simulink library "powerlib_modelsV2"  (Simulink 6.0)
settings: Solver=ode45  SolverMode=SingleTasking  StartTime=0.0  StopTime=10.0  RelTol=1e-3
values from neighbouring files (symbols this model uses):
  Ts = get(handles.edit1,'string')    [powergui.m]
undefined symbols (not defined in the file or in its folder): A, Ac, B, Bc, C, Cc, Cs, Current, damp, Dc, Dd, DiscIntNeverNeededParam, dref, dwo, exc, F, fb, gate, GH, GHd, GI, GId, GL, GLd, H, HT, hyd, ib, ib2, io, isfinite, j, K, Kd, Kg, L, Lad, Laq, lim, LIM, Ll, Llfd, Llkd, Llkq1, Llkq2, Llr, Lls, LowerFlux, N, N2, Nb, Nb2, nb_arm, p, Par_HarmoA_pu, Par_HarmoB_pu, Par_Timing_Harmo, Par_Timing_Variation, Par_Vps, Pb ... (+57)
libraries: powerlib_extras x14
(part 2 of 11)

== system powerlib_modelsV2/Discrete ==
  3_Phase_Prog_Source : Subsystem  mask(Discrete 3-phase Programmable Source){Par_Vps_LLrms=[1.01 -20  60], VariationEntity=Amplitude, VariationType=Step, VariationStep=-0.5, VariationRate=10, VariationMag=0.3, VariationFreq=2, Par_Timing_Variation=[0.1 1.2], SinglePhase=off, Yampli=[1 0.8 1.2 1.0], Xtime=[0 0.1 0.15 0.2], HarmonicGeneration=off, Par_HarmoA_pu=[3 0.2 -25 0], Par_HarmoB_pu=[2 0.15 35 2], Par_Timing_Harmo=[0.05  3], Ts=50e-6}
      mask prompts: Par_Vps_LLrms "Positive-sequence: [ Amplitude  Phase(degrees)   Freq. (Hz) ]"; VariationEntity "Time variation of:"; VariationType "Type of variation:"; VariationStep "Step magnitude:"; VariationRate "Rate of change (value/s):"; VariationMag "Amplitude of the modulation:"; VariationFreq "Frequency of the modulation(Hz):"; Par_Timing_Variation "Variation timing (s) : [ Start   End ]"; SinglePhase "1-phase only"; Yampli "Amplitude values:"; Xtime "Time values:"; HarmonicGeneration "Harmonic generation:"; Par_HarmoA_pu "A:  [ Order(n)   Amplitude  Phase(degrees)  Seq(0, 1 or 2) ]"; Par_HarmoB_pu "B:  [ Order(n)   Amplitude  Phase(degrees)  Seq(0, 1 or 2) ]"; Par_Timing_Harmo "Harmonic timing (s) : [ Start   End ]"; Ts "Sample time:"
      mask help: Use this discrete block to generate a set of three-phase sinusoidal voltages or currents a, b and c. Time variation for the amplitude, phase and frequency of the fundamental can be pre-programmed. In addition, two harmonics can be surimposed on the fundamental.
      mask init:
      | % Conversion of pos. seq.amplitude from Ph-Ph rms voltage to Ph-G peak
      | Par_Vps=Par_Vps_LLrms;
      | Par_Vps(1)=Par_Vps(1)*sqrt(2/3);
      | Mag_Vps=Par_Vps(1);
      | Phase_Vps=Par_Vps(2);
      | Freq_Vps=Par_Vps(3);
      | % Conversion of harmonic amplitudes from pu to Ph-G peak volt
      | Par_HarmoA=Par_HarmoA_pu;
      | Par_HarmoB=Par_HarmoB_pu;
      | Par_HarmoA(2)=Par_HarmoA(2)*Mag_Vps;
      | Par_HarmoB(2)=Par_HarmoB(2)*Mag_Vps;
      | % Conversion of amplitude variation from pu to Ph-G peak volt
      | if VariationEntity==2
      | 	VariationStep=VariationStep*Mag_Vps;
      | 	VariationRate=VariationRate*Mag_Vps;
      | 	VariationMag=VariationMag*Mag_Vps;
      | 	Yampli=Yampli*Mag_Vps;
      | end
      | 
      | Ton_Variation=Par_Timing_Variation(1);
      | Toff_Variation=Par_Timing_Variation(2);
      | n_HarmoA=Par_HarmoA(1);
      | Mag_HarmoA=Par_HarmoA(2);
      | Phase_HarmoA=Par_HarmoA(3);
      | Seq_HarmoA=Par_HarmoA(4);
      | if n_HarmoA==0
      |     Phase_HarmoA=90;
      |     Seq_HarmoA=0;
      | end
      | n_HarmoB=Par_HarmoB(1);
      | Mag_HarmoB=Par_HarmoB(2);
      | Phase_HarmoB=Par_HarmoB(3);
      | Seq_HarmoB=Par_HarmoB(4);
      | if n_HarmoB==0
      |     Phase_HarmoB=90;
      |     Seq_HarmoB=0;
      | end
      | Ton_Harmo=Par_Timing_Harmo(1);
      | Toff_Harmo=Par_Timing_Harmo(2);
      | if Xtime(1)~=0,
      | Xtime=[0 Xtime];
      | Yampli=[0 Yampli];
      | end
      | n=length(Xtime); vec_dt= [Xtime,0] - [0,Xtime] ; vec_dt=vec_dt(2:n);
      mask StyleString: edit,popup(None|Amplitude|Phase|Frequency),popup(Step|Ramp|Modulation|Table of time-amplitude pairs),edit,edit,edit,edit,edit,checkbox,edit,edit,checkbox,edit,edit,edit,edit
      mask CallbackString: |parametres=get_param(gcb,'MaskValues');p2=parametres{2};p3=parametres{3};p12=parametres{12};if strcmp(p3,'Step');param4='on';param5='off';param6='off';param7='off';param8='on';param9='off';param10='off';param11='off';elseif strcmp(p3,'Ramp');param4='off';param5='on';param6='off';param7='off';param8='on';param9='off';param10='off';param11='off';elseif strcmp(p3,'Modulation');param4='off';param5='off';param6='on';param7='on';param8='on';param9='off';param10='off';param11='off';else;param4='off';param5='off';param6='off';param7='off';param8='off';param9='on';param10='on';param11='on';end;if strcmp(p2,'None');param3='off';param4='off';param5='off';param6='off';param7='off';param8='off';param9='off';param10='off';param11='off';else;param3='on';end;if strcmp(p12,'on');param13='on';param14='on';param15='on';else;param13='off';param14='off';param15='off';end;visible={'on','on',param3,param4,param5,param6,param7,param8,param9,param10,param11,'on',param13,param14,param15,'on'};set_param(gcb,'MaskVisibilities',visible)|parametres=get_param(gcb,'MaskValues');p2=parametres{2};p3=parametres{3};p12=parametres{12};if strcmp(p3,'Step');param4='on';param5='off';param6='off';param7='off';param8='on';param9='off';param10='off';param11='off';elseif strcmp(p3,'Ramp');param4='off';param5='on';param6='off';param7='off';param8='on';param9='off';param10='off';param11='off';elseif strcmp(p3,'Modulation');param4='off';param5='off';param6='on';param7='on';param8='on';param9='off';param10='off';param11='off';else;param4='off';param5='off';param6='off';param7='off';param8='off';param9='on';param10='on';param11='on';end;if strcmp(p2,'None');param3='off';param4='off';param5='off';param6='off';param7='off';param8='off';param9='off';param10='off';param11='off';else;param3='on';end;if strcmp(p12,'on');param13='on';param14='on';param15='on';else;param13='off';param14='off';param15='off';end;visible={'on','on',param3,param4,param5,param6,param7,param8,param9,param10,param11,'on',param13,param14,param15,'on'};set_param(gcb,'MaskVisibilities',visible)|||||||||parametres=get_param(gcb,'MaskValues');p2=parametres{2};p3=parametres{3};p12=parametres{12};if strcmp(p3,'Step');param4='on';param5='off';param6='off';param7='off';param8='on';param9='off';param10='off';param11='off';elseif strcmp(p3,'Ramp');param4='off';param5='on';param6='off';param7='off';param8='on';param9='off';param10='off';param11='off';elseif strcmp(p3,'Modulation');param4='off';param5='off';param6='on';param7='on';param8='on';param9='off';param10='off';param11='off';else;param4='off';param5='off';param6='off';param7='off';param8='off';param9='on';param10='on';param11='on';end;if strcmp(p2,'None');param3='off';param4='off';param5='off';param6='off';param7='off';param8='off';param9='off';param10='off';param11='off';else;param3='on';end;if strcmp(p12,'on');param13='on';param14='on';param15='on';else;param13='off';param14='off';param15='off';end;visible={'on','on',param3,param4,param5,param6,param7,param8,param9,param10,param11,'on',param13,param14,param15,'on'};set_param(gcb,'MaskVisibilities',visible)||||
  3_phase_source : Subsystem  mask{A=1, P=0, F=60, Ts=0}
      mask prompts: A "Amplitude"; P "Phase (of phase A)"; F "Frequency"; Ts "Sample Time"
  Dynamic_Load : Subsystem  mask(Discrete 3-Phase Dynamic Load ){Vfnom=[ 500e3 60 ], PQ_0=[ 50e6 25e6]*0.8504^2, V0=[0.8504  -41.9 ], PQext=off, n=[1 2], Tpq=[0  0  0  0], Vmin=0.7, Reserved=0, Ts=Ts}
      mask prompts: Vfnom "Nominal L-L voltage and freqency  [Vn(Vrms) fn(Hz)]:"; PQ_0 "Active & reactive power at initial voltage [Po(W) Qo(var)]:"; V0 "Initial positive-sequence voltage Vo [Mag(pu) Phase (deg.)]:"; PQext "External control of PQ"; n "Parameters [ np  nq ]:"; Tpq "Time constants [Tp1 Tp2 Tq1 Tq2]  (s):"; Vmin "Minimum voltage Vmin (pu):"; Ts "Sample time (s):"
      mask help:
      | This block implements a three-phase, three-wire dynamic load whose active  power P and reactive power Q vary as function of positive-sequence voltage. Negative- and zero-sequence currents are not simulated. The three load currents are therefore balanced, even under unbalanced load voltage conditions.
      |
      |   If V>Vmin, P and Q vary as follows:
      |        P=Po*(V/Vo)^np*(1+Tp1s)/(1+Tp2s)
      |        Q=Qo*(V/Vo)^nq*(1+Tq1s)/(1+Tq2s)
      | where:
      | Po, Qo : Active and reactive powers at specified voltage Vo
      |   V :        Positive-sequence voltage
      |   Vmin :  Minimum voltage below which load impedance
      |                is kept constant (np=nq=2)
      | np,nq :    Exponents (usually comprised between 1 and 3)
      |                controlling the nature of the load.
      | Tp1,Tp2 : Time constants controlling the dynamics of P
      | Tq1,Tq2 : Time constants controlling the dynamics of Q
      |
      | For example, specify  np=nq=1 for a constant current load; np=nq=2  for a  constant impedance load.
      |
      | Check 'External control of PQ'  to control power from a vectorized signal  [P Q] connected to input  4.
      | The m output returns a vector of 3 signals [V(pu) P(W) Q (var)].
      mask init: same as powerlib_modelsV2/Continuous/Dynamic_Load
      mask CallbackString: |||parametres=get_param(gcb,'MaskValues');p4=parametres{4};if strcmp(p4,'on');param5='off';param6='off';param7='off';else ;param5='on';param6='on';param7='on';end;visible={'on','on','on','on',param5,param6,param7,'on','on'};set_param(gcb,'MaskVisibilities',visible)|||||
  Excitation_System : Subsystem  mask(Discrete Excitation System){tr=tr, reg=reg, exc=exc, tgr=tgr, damp=damp, sat=sat, lim=lim, v0=v0, Ts=50e-6}
      mask prompts: tr "Low-pass filter time constant Tr(s):"; reg "Regulator gain and time constant [ Ka()  Ta(s) ]:"; exc "Exciter  [ Ke()  Te(s) ]:"; tgr "Transient gain reduction [ Tb(s)  Tc(s) ]:"; damp "Damping filter gain and time constant  [ Kf()  Tf(s)  ]:"; sat "Field saturation parameters [ A, B ]:"; lim "Regulator output limits and gain [ Efmin, Efmax (p.u.), Kp() ]:"; v0 "Initial values of terminal voltage  and field voltage [ Vt0 (pu) Vf0(pu) ] :"; Ts "Sample time:"
      mask help:
      | Implements an discrete IEEE type 1 synchronous machine voltage regulator combined to an exciter. This block uses the dq components of terminal voltage (Synchronous Machine block, measurement ouputs 9 and 10).
      |
      | 1st input: desired stator terminal voltage (p.u.);
      | 2nd input: vd component of the terminal voltage (p.u.);
      | 3rd input: vq component of the terminal voltage (p.u.);
      | 4th input: stabilization voltage from user-supplied
      |                  power system stabilizer (p.u.);
      |
      | output: field voltage vfd to be applied to the
      |              Synchronous Machine block's 2nd input (p.u.).
      mask init:
      | ka=reg(1);ta=reg(2);ke=exc(1);te=exc(2);tb=tgr(1);tc=tgr(2);kf=damp(1);tf=damp(2);efmin=lim(1);efmax=lim(2);a=sat(1);b=sat(2);kp=lim(3);
      | if te==0,
      | te=1e-6;
      | end
      mask Help: web(psbhelp);
  GTO-IGBT Bridge : Subsystem  mask(GTO & IGBT Bridge Logic){nb_arm=3, Tf=0, Tt=0, Cs=Inf, VFs=[0 0], Rsw=1, Ts=1}
      mask prompts: nb_arm "Number of bridge arms (1,2 or 3)"; Tf "Curent 10% fall time Tf (s) :"; Tt "Current tail time Tt (s) :"; Cs "Snubber Capacitance Cs (F):"; VFs "Forward Voltages [ Vf  Vfd ]"; Rsw "Device resistance"; Ts "Time step Ts (s) :"
      mask help:
      | Generates the switch status ( 0 or 1) and the tail currents for a forced-commutated two- level bridge using GTO/Diode or IGBT/Diode pairs.
      | Specify  3 arms (6 switches) for 3 phase bridge, 2 arms for 4 switches, or 1 arm.
      | To turn-off the tail current, specify Tf=0 and Tt=0.
      mask init:
      | Vf=VFs(1);
      | Vfd=VFs(2);
      | nb_switch=nb_arm*2;
      | if nb_arm==1,
      |    Selec_Diode=[2 1];
      | elseif nb_arm==2,
      |    Selec_Diode=[2 1 4 3];
      | elseif nb_arm==3,
      |    Selec_Diode=[2 1 4 3 6 5];
      | end
  HTG : Subsystem  mask(Discrete Hydraulic Turbine and Governor){sm=sm, gate=gate, reg=reg, hyd=hyd, dref=dref, po=po, Ts=50e-6}
      mask prompts: sm "Servo-motor [ Ka()  Ta(sec) ]:"; gate "Gate opening limits [ gmin,gmax(pu)    vgmin,vgmax(pu/s) ]:"; reg "Permanent droop and regulator  [ Rp() Kp() Ki() Kd() Td(s) ]:"; hyd "Hydraulic turbine [ beta()  Tw(sec) ]:"; dref "Droop reference (0=power error, 1=gate opening):"; po "Initial mechanical power (pu):"; Ts "Sample time:"
      mask help:
      | Implements a discrete hydraulic turbine combined to a discrete PID governor system.
      |
      | 1st input: desired speed (p.u.);
      | 2nd input: desired electrical power (p.u.);
      | 3rd input: synchronous machine's actual speed (p.u., measurement output 13 of SM block);
      | 4th input: synchronous machine's actual electrical power (p.u., measurement output 14 of SM block);
      | 5th input: synchronous machine's actual speed deviation with respect to nominal (%, measurement output 15 of SM block);
      |
      | 1st output: mechanical power to be applied to the Synchronous Machine block's 1st input (p.u.);
      | 2nd output: gate opening (p.u.).
      mask init:
      | ka=sm(1);ta=sm(2);gmin=gate(1);gmax=gate(2);vgmin=gate(3);vgmax=gate(4);Rp=reg(1);kp=reg(2);ki=reg(3);kd=reg(4);td=reg(5);beta=hyd(1);tw=hyd(2);go=po*(gmax-gmin);
      mask Help: web(psbhelp);
  Impedance Measurement : Subsystem
      mask Type: Impedance Measurement model
      mask Description: The impedance Measurement block injects a null current in the circuit.
  MBPSS : Subsystem  mask(MB-PSS ){OperationMode=Detailed settings, Kg=Kg, GL=GL, GI=GI, GH=GH, GLd=GLd, TcLF=TcLF, GId=GId, TcIF=TcIF, GHd=GHd, TcHF=TcHF, LIM=LIM, Plot_On=off, MagdB_On=off, FreqRange=logspace(-2,2,500), Ts=50e-6}
      mask prompts: OperationMode "Mode of operation:"; Kg "Global gain:"; GL "Low frequency band: [ FL(Hz), KL ]"; GI "Intermediate frequency band: [ FI(Hz), KI ]"; GH "High frequency band: [ FH(Hz), KH ]"; GLd "Low frequency gains: [ KL1, KL2, KL ]"; TcLF "Low frequency  time constants (s):"; GId "Intermediate frequency gains: [ KI1, KI2, KI ]"; TcIF "Intermediate frequency time constants (s):"; GHd "High frequency gains: [ KH1, KH2, KH ]"; TcHF "High frequency time constants (s):"; LIM "Signals Limits(VLmax,VImax,VHmax,VSmax)"; Plot_On "Plot frequency response"; MagdB_On "Magnitude in dB"; FreqRange "Frequency range (Hz):"
      mask help:
      | This block implements a Multi-band Power System Stabilizer (MB-PSS). Two operation modes are available: Detailed setting and simplified setting (IEEE Std 421.5).
      |
      | Input (dw): Synchronous machine speed deviation with respect to nominal (pu).
      | Output: stabilization voltage (pu).
      |
      | Note:
      | When "Detailed settings" is used, the low(L)-, intermediate(I)- and high(H)-frequency time constants must be given in the following order:
      | Tx1 to Tx12 followed by Kx11 and Kx17 (where x=L, I or H). Look under mask to see in which transfer functions these time constants are used.
      mask init:
      | Detailed=0;
      | if OperationMode==2,
      | Detailed=1;
      | Kg=1;
      | KL1=GLd(1);KL2=GLd(:,2);KL=GLd(3);
      | TL1=TcLF(1);TL2=TcLF(2);TL3=TcLF(3);TL4=TcLF(4);
      | TL5=TcLF(5);TL6=TcLF(6);TL7=TcLF(7);TL8=TcLF(8);
      | TL9=TcLF(9);TL10=TcLF(10);TL11=TcLF(11);TL12=TcLF(12);
      | KL11=TcLF(13);KL17=TcLF(14);
      | KI1=GId(1);KI2=GId(:,2);KI=GId(3);
      | TI1=TcIF(1);TI2=TcIF(2);TI3=TcIF(3);TI4=TcIF(4);
      | TI5=TcIF(5);TI6=TcIF(6);TI7=TcIF(7);TI8=TcIF(8);
      | TI9=TcIF(9);TI10=TcIF(10);TI11=TcIF(11);TI12=TcIF(12);
      | KI11=TcIF(13);KI17=TcIF(14);
      | KH1=GHd(1);KH2=GHd(:,2);KH=GHd(3);
      | TH1=TcHF(1);TH2=TcHF(2);TH3=TcHF(3);TH4=TcHF(4);
      | TH5=TcHF(5);TH6=TcHF(6);TH7=TcHF(7);TH8=TcHF(8);
      | TH9=TcHF(9);TH10=TcHF(10);TH11=TcHF(11);TH12=TcHF(12);
      | KH11=TcHF(13);KH17=TcHF(14);
      | else
      | %
      | R=1.2;K=(R*R+R)/(R*R-2*R+1);KL1=K;KL2=K;KI1=K;KI2=K;KH1=K;KH2=K;
      | TL2=1/(2*pi*GL(1)*sqrt(R));KL=GL(2);TL1=TL2/R;TL7=TL2;TL8=TL7*R;
      | %
      | TI2=1/(2*pi*GI(1)*sqrt(R));KI=GI(2);TI1=TI2/R;TI7=TI2;TI8=TI7*R;
      | TH2=1/(2*pi*GH(1)*sqrt(R));KH=GH(2);TH1=TH2/R;TH7=TH2;TH8=TH7*R;
      | %
      | TL3=0;TL4=0;TL5=0;TL6=0;TL9=0;TL10=0;TL11=0;TL12=0;
      | TI3=0;TI4=0;TI5=0;TI6=0;TI9=0;TI10=0;TI11=0;TI12=0;
      | TH3=0;TH4=0;TH5=0;TH6=0;TH9=0;TH10=0;TH11=0;TH12=0;
      | KL11=1;KL17=1;KI11=1;KI17=1;KH11=1;KH17=1;
      | end
      | LIM_VL=LIM(1);LIM_VI=LIM(2);LIM_VH=LIM(3);LIM_VS=LIM(4);
      | %
      | % LF Transfer function
      | numLF1=[TL1 KL11];
      | denLF1=[TL2 1];
      | sysLF1=tf(numLF1,denLF1);
      | numLF2=[TL3 1];
      | denLF2=[TL4 1];
      | sysLF2=tf(numLF2,denLF2);
      | numLF3=[TL5 1];
      | denLF3=[TL6 1];
      | sysLF3=tf(numLF3,denLF3);
      | numLF4=[TL7 KL17];
      | denLF4=[TL8 1];
      | sysLF4=tf(numLF4,denLF4);
      | numLF5=[TL9 1];
      | denLF5=[TL10 1];
      | sysLF5=tf(numLF5,denLF5);
      | numLF6=[TL11 1];
      | denLF6=[TL12 1];
      | sysLF6=tf(numLF6,denLF6);
      | %
      | sysLF=Kg*KL*((KL1*sysLF1*sysLF2*sysLF3) - (KL2*sysLF4*sysLF5*sysLF6));
      | %
      | %
      | % IF transfer function
      | numIF1=[TI1 KI11];
      | denIF1=[TI2 1];
      | sysIF1=tf(numIF1,denIF1);
      | numIF2=[TI3 1];
      | denIF2=[TI4 1];
      | sysIF2=tf(numIF2,denIF2);
      | numIF3=[TI5 1];
      | denIF3=[TI6 1];
      | sysIF3=tf(numIF3,denIF3);
      | numIF4=[TI7 KI17];
      | denIF4=[TI8 1];
      | sysIF4=tf(numIF4,denIF4);
      | numIF5=[TI9 1];
      | denIF5=[TI10 1];
      | sysIF5=tf(numIF5,denIF5);
      | numIF6=[TI11 1];
      | denIF6=[TI12 1];
      | sysIF6=tf(numIF6,denIF6);
      | %
      | sysIF=Kg*KI*((KI1*sysIF1*sysIF2*sysIF3) - (KI2*sysIF4*sysIF5*sysIF6));
      | %
      | %
      | % HF transfer function
      | numHF1=[TH1 KH11];
      | denHF1=[TH2 1];
      | sysHF1=tf(numHF1,denHF1);
      | numHF2=[TH3 1];
      | denHF2=[TH4 1];
      | sysHF2=tf(numHF2,denHF2);
      | numHF3=[TH5 1];
      | denHF3=[TH6 1];
      | sysHF3=tf(numHF3,denHF3);
      | numHF4=[TH7 KH17];
      | denHF4=[TH8 1];
      | sysHF4=tf(numHF4,denHF4);
      | numHF5=[TH9 1];
      | denHF5=[TH10 1];
      | sysHF5=tf(numHF5,denHF5);
      | numHF6=[TH11 1];
      | denHF6=[TH12 1];
      | sysHF6=tf(numHF6,denHF6);
      | %
      | sysHF=Kg*KH*((KH1*sysHF1*sysHF2*sysHF3) - (KH2*sysHF4*sysHF5*sysHF6));
      | %
      | %
      | % Input filter LIF
      | numLIFin=[1.759e-3 1];
      | denLIFin=[1.2739e-4 1.7823e-2 1];
      | sysLIFin=tf(numLIFin,denLIFin);
      | % Input filter HF
      | numHFin=[80 0 0];
      | denHFin=[1 82 161 80];
      | sysHFin=tf(numHFin,denHFin);
      | %
      | % Global transfer function:
      | sysL=sysLIFin*sysLF;
      | sysI=sysLIFin*sysIF;
      | sysH=sysHFin*sysHF;
      | sysG=sysL+sysI + sysH;
      | %
      | % Plot frequency response:
      | if Plot_On==1,
      |     w=2*pi*FreqRange;
      |     [MagL,PhaseL]=bode(sysL,w);
      |     [MagI,PhaseI]=bode(sysI,w);
      |     [MagH,PhaseH]=bode(sysH,w);
      |     [MagG,PhaseG]=bode(sysG,w);
      |     subplot(2,1,1)
      |      if  MagdB_On==1,
      |         YL= 20*log10(squeeze(MagL)) ;
      |         YI= 20*log10(squeeze(MagI)) ;
      |         YH= 20*log10(squeeze(MagH)) ;
      |         YG= 20*log10(squeeze(MagG)) ;
      |          strLabel='dB';
      | else
      | YL=squeeze(MagL);
      | YI=squeeze(MagI);
      | YH=squeeze(MagH);
      | YG=squeeze(MagG);
      | strLabel='pu/pu';
      | end
      | semilogx(FreqRange,YL,'m',FreqRange,YI,'g',FreqRange,YH,'b',FreqRange,YG,'r')
      | ylabel(strLabel);grid;
      | legend('LF band','IF band','HF band','Global',2);
      | title('MB-PSS Frequency Response');
      |  subplot(2,1,2);
      | semilogx(FreqRange,rem(squeeze(PhaseL),360),'m',FreqRange,rem(squeeze(PhaseI),360),'g',FreqRange,rem(squeeze(PhaseH),360),'b',FreqRange,rem(squeeze(PhaseG),360),'r');
      | ylabel('Degrees');grid;
      | xlabel('Frequency (Hz)');
      | end
      mask StyleString: popup(Simplified settings|Detailed settings),edit,edit,edit,edit,edit,edit,edit,edit,edit,edit,edit,checkbox,checkbox,edit,edit
      mask CallbackString: parametres=get_param(gcb,'MaskValues');p1=parametres{1};p13=parametres{13};if strcmp(p1,'Detailed settings');param2='off';param3='off';param4='off';param5='off';param6='on';param7='on';param8='on';param9='on';param10='on';param11='on';else;param2='on';param3='on';param4='on';param5='on';param6='off';param7='off';param8='off';param9='off';param10='off';param11='off';end;if strcmp(p13,'on');param14='on';param15='on';else;param14='off';param15='off';end;visible={'on',param2,param3,param4,param5,param6,param7,param8,param9,param10,param11,'on','on',param14,param15,'on'};set_param(gcb,'MaskVisibilities',visible)||||||||||||parametres=get_param(gcb,'MaskValues');p1=parametres{1};p13=parametres{13};if strcmp(p1,'Detailed settings');param2='off';param3='off';param4='off';param5='off';param6='on';param7='on';param8='on';param9='on';param10='on';param11='on';else;param2='on';param3='on';param4='on';param5='on';param6='off';param7='off';param8='off';param9='off';param10='off';param11='off';end;if strcmp(p13,'on');param14='on';param15='on';else;param14='off';param15='off';end;visible={'on',param2,param3,param4,param5,param6,param7,param8,param9,param10,param11,'on','on',param14,param15,'on'};set_param(gcb,'MaskVisibilities',visible)|||
  PM_synchronous_machine : Subsystem  mask(PM Synchronous Machine Model){R=0.6, L=[ 1.4e-3, 2.8e-3], lam=0.1, mec=[ 1.1e-3, 1.4e-3,  4 ], Ts=1}
      mask prompts: R "Resistance R(ohm):"; L "Inductances [ Ld(H) Lq(H) ]:"; lam "Flux induced by magnets (Wb):"; mec "Inertia, friction factor and pairs of poles [ J(kg.m^2)  F(N.m.s)  p() ]:"; Ts "Sample Time (s):"
      mask help:
      | Implements a 3-phase permanent magnet synchronous machine with sinusoidal flux distribution. The machine is modelled in the qd rotor reference frame. Stator windings are connected in wye to an internal neutral point.
      |
      | First 3 inputs: Machine terminals =  phases a, b and c
      | 4th input:  Simulink signal = mechanical torque (N.m)
      |                    (>0 for motor mode,<0 for generator mode)
      |
      | output: Simulink measurement output = vector (10x1) containing
      |              (all currents flowing into machine):
      |   1-3 : Stator line currents ia, ib, ic (A)
      |   4-5 : Stator currents iq, id (A)
      |   6-7 : Stator voltages vq, vd (V)
      |   8     : Rotor electrical speed we (rad/s)
      |   9     : Rotor electrical angle theta (deg)
      |   10   : Electromagnetic torque Te (N.m)
      mask init:
      | Ld=L(1);Lq=L(2);J=mec(1);F=mec(2);p=mec(3);sqrt3=sqrt(3);one_third=1/3;
  PSS : Subsystem  mask(Generic PSS){Tsensor=Tsensor, K=K, Twashout=Twashout, Tleadlag1=Tleadlag1, Tleadlag2=Tleadlag2, VSlimits=VSlimits, Vinit=Vinit, Plot_On=off, MagdB_On=on, FreqRange=logspace(-2,2,500), Ts=50e-6}
      mask prompts: Tsensor "Sensor time constant:"; K "Gain:"; Twashout "Wash-out time constant:"; Tleadlag1 "Lead-lag #1 time constants: [ Tnum Tden ]"; Tleadlag2 "Leag-lag #2 time constants: [ Tnum Tden ]"; VSlimits "Output limits: [ VSmin VSmax ]"; Vinit "Initial input:"; Plot_On "Plot frequency response"; MagdB_On "Magnitude in dB"; FreqRange "Frequency range (Hz):"
      mask help:
      | This block implements a generic Power System Stabilizer (PSS).
      |
      | Input (In): Synchronous machine speed deviation with respect to nominal (dw in pu) or acceleration power (Pa=Pm-Pe in pu).
      | Output (VS): stabilization voltage (pu).
      |
      | Look under mask to see how the various transfer functions are connected.
      mask init:
      | T1n=Tleadlag1(1);
      | T1d=Tleadlag1(2);
      | T2n=Tleadlag2(1);
      | T2d=Tleadlag2(2);
      | %
      | if Plot_On==1,
      | % Compute global system (sysG):
      | numS=[1];
      | denS=[Tsensor 1];
      | sysS=tf(numS,denS);
      | numW=[Twashout 0];
      | denW=[Twashout 1];
      | sysW=tf(numW,denW);
      | numL1=[T1n 1];
      | denL1=[T1d 1];
      | sysL1=tf(numL1,denL1);
      | numL2=[T2n 1];
      | denL2=[T2d 1];
      | sysL2=tf(numL2,denL2);
      | sysG=sysS*K*sysW*sysL1*sysL2;
      | %
      | % Plot response:
      | w=2*pi*FreqRange;
      | [Mag,Pha]=bode(sysG,w);
      | subplot(2,1,1)
      | if  MagdB_On==1,
      | Y= 20*log10(squeeze(Mag)) ;
      | strLabel='dB';
      | else
      | Y=squeeze(Mag);
      | strLabel='pu/pu';
      | end
      | %
      | semilogx(FreqRange,Y)
      | ylabel(strLabel);grid;
      | title('PSS Frequency Response');
      | subplot(2,1,2);
      | semilogx(FreqRange,rem(squeeze(Pha),360))
      | ylabel('Degrees');grid;
      | xlabel('Frequency (Hz)');
      | end
      mask CallbackString: |||||||parametres=get_param(gcb,'MaskValues');p8=parametres{8};if strcmp(p8,'on');param9='on';param10='on';else;param9='off';param10='off';end;visible={'on','on','on','on','on','on','on','on',param9,param10,'on'};set_param(gcb,'MaskVisibilities',visible)|||
  Three-Level Bridge : Subsystem  mask(Three-level Bridge Logic){nb_arm=1, Cs=inf, Par_Vf=[0 0], Ron=1, Ts=1}
      mask prompts: nb_arm "Number of bridge arms (1,2 or 3)"; Cs "Snubber capacitance Cs (F):"; Par_Vf "Forward Voltages [ Vf  Vfd ]:"; Ron "Internal resistance Ron (Ohms):"; Ts "Sample time"
      mask init:
      | if nb_arm==1,
      |    StatusElements=[1 2 3];
      | elseif nb_arm==2,
      |    StatusElements=[1 2 5 3 4 6];
      | elseif nb_arm==3,
      |    StatusElements=[1 2 7 3 4 8 5 6 9];
      | end
  asynchronous_machine : Subsystem  mask(Asynchronous Machine Model){rotType=Wound, ctrl=Rotor, nom=[2.2380e+03  2.2000e+02  6.0000e+01], sta=[2.0114e-02  3.4865e-02], rot=[3.7732e-02  3.4865e-02], Lm=[1.2082e+00], mec=[7.0650e-01  0.0000e+00  2.0000e+00], ini=[1.0000e+00  0.0000e+00  0.0000e+00  0.0000e+00  0.0000e+00  0.0000e+00  0.0000e+00  0.0000e+00], iounits=on, Ts=1}
      mask prompts: rotType "Rotor type:"; ctrl "Reference frame:"; nom "Nom. power,L-L volt. and freq. [ Pn(VA),Vn(Vrms),fn(Hz) ]:"; sta "Stator [ Rs,Lls (p.u.) ]:"; rot "Rotor [ Rr',Llr' (p.u.) ]:"; Lm "Magnetizing inductance Lm (p.u.):"; mec "Inertia constant,friction factor and pairs of poles [ H(s)  F(p.u.)  p() ]:"; ini "Initial conditions [ s()  th(deg)   isa,isb,isc(p.u.)   pha,phb,phc(deg) ]:"; iounits "I/O units (check for S.I., otherwise p.u.)"; Ts "Sample Time Ts (s):"
      mask help: Implements a three-phase asynchronous machine (wound rotor or squirrel cage) modelled in the dq rotor reference frame. Stator and rotor windings are connected in wye to an internal neutral point. Press help for inputs and outputs description.
      mask init: same as powerlib_modelsV2/Continuous/asynchronous_machine
      mask Help: First 3 inputs: Stator terminals = phases a, b and c; 4th input: Simulink signal = Mechanical torque applied to the shaft (p.u., >0 for motor mode, <0 for generator mode); First 3 outputs: Rotor terminals = phases a, b and c; 4th output: Simulink measurement output = vector (20x1) containing the following (all currents flowing into the machine): [1-3] : Rotor line currents ira, irb and irc; [4-5] : Rotor currents iqr and idr; [6-7] : Rotor fluxes phiqr and  phidr; [8-9] : Rotor voltages vqr and vdr; [10-12] : Stator line currents isa, isb, isc; [13-14] : Stator currents iqs and ids; [15-16] : Stator fluxes phiqs and  phids; [17-18] : Stator voltages vqs and vds; [19] : Rotor speed wm; [20 ]: Electromagnetic torque Te. Units of output measurement depend on checkbox in block's dialog box.
      mask StyleString: popup(Wound|Squirrel-cage),popup(Rotor|Stationary|Synchronous),edit,edit,edit,edit,edit,edit,checkbox,edit
  breaker : Subsystem  mask(Breaker Model){Nsw=1, istate=0, Rsw=1, Ts=1}
      mask prompts: Nsw "Number of breaker"; istate "Initial state"; Rsw "Breaker resistances"; Ts "Sample time (s):"
      mask help: Simulink model for the Breaker block.
  detailed_thyristor (logical) : Subsystem  mask(thyristors logic model){Nsw=1, Vf=0, Rsw=1, Ts=1}
      mask prompts: Nsw "Number of thyristors"; Vf "Forward voltage Vf (V):"; Rsw "Thyristor resistances"; Ts "Sample time (s):"
  diode (logical) : Subsystem  mask(Diode logic model){Nsw=1, Vf=0, Rsw=1, Ts=1}
      mask prompts: Nsw "Number of diodes"; Vf "Forward Voltage Vf (V):"; Rsw "Diode resistances"; Ts "Sample time (s):"
  distributed_param_line : Subsystem  mask(Distributed Parameter Line Model){nphase=3, f=60, ri=[0.01273 0.3864], li=[0.9337e-3  4.1264e-3], ci=[12.74e-9 7.751e-9], long=100, V1_init=[0 0 0 0; 0.0001244 0 0 0; 0.0002488 0 0 0; 0.0003733 0 0 0; 0.0004977 0 0 0; 0.0006221 0 0 0], V2_init=[0 0 0 0; 0.0001244 0 0 0; 0.0002488 0 0 0; 0.0003733 0 0 0; 0.0004977 0 0 0; 0.0006221 0 0 0], I1_init=[0 0 0 0; 0.0001244 0 0 0; 0.0002488 0 0 0; 0.0003733 0 0 0; 0.0004977 0 0 0; 0.0006221 0 0 0], I2_init=[0 0 0 0; 0.0001244 0 0 0; 0.0002488 0 0 0; 0.0003733 0 0 0; 0.0004977 0 0 0; 0.0006221 0 0 0], time_init=0}
      mask prompts: nphase "Number of phases"; f "Frequency used for R L C specification (Hz)"; ri "R [3*3 matrix] or [R0 R1] (ohms/km)"; li "L [3*3matrix ] or [L0 L1] (H/km)"; ci "C [3*3matrix] or [C0 C1] (F/km)"; long "Line length (km)"; time_init "time delay init"
      mask help: N phases distributed parameters line with losses
      mask init:
      | [Zm,R,v,Ti]=powericonV2('Distributed Parameter Line Model',nphase,f,ri,li,ci);to=long./v;Rt4=R*long/4;h=(Zm-Rt4)./(Zm+Rt4);
      mask Help:
      | Multiphase distributed parameter line.  For symetrical or asymetrical lines, R L and C parameters are specified by NxN matrices
      | For 2-phase, 3-phase and six-phase symetrical lines, R L C parameters can be also specified by sequence component vectors:  ie [R0 R1] for 2 and 3 phase line or [R1 R0 R0m] for a six-phase line representing two identical coupled 3-phase circuits.
  hysteresis_transformer : Subsystem  mask(Saturable transformer model){isat=[-734.846922834953 0 0 734.846922834953], phisat=[-1624.36833590349 -1191.20344632923 1191.20344632923 1624.36833590349], fluxinit=0, initialslope=+1, matfile='hysteresis', indice=1, fluxbase=1082.91222393566, currentbase=734.846922834953, Ts=Ts}
      mask prompts: isat "Saturation current:"; phisat "Flux saturation:"; fluxinit "Initial flux:"; initialslope "pente initiale du flux initial"; matfile "Mat file"; indice "Transfo no:"; fluxbase "Base flux"; currentbase "Base current"; Ts "Sample time Ts(sec):"
      mask help:
      | Models the saturation of a three winding saturable transformer.
      |
      | The saturation characteristic should be given in increasing order starting with current-flux pair (0,0). Only positive part of the characteristic must be entered. If the initial flux parameter (phi0) is not declared, the flux will be initialized automatically according to the steady-state voltage across the magnetizing branch. Set winding no.3 parameters to zero to implement a two winding transformer.
      mask init:
      | [fb,ib,Tolerances,HT,UpperFlux,LowerFlux,Current] = powericonV2('inithysteresis',matfile,1,fluxbase,currentbase);
  ideal_switch : Subsystem  mask(Switch logic model){Nsw=1, Rsw=1, Ts=1}
      mask prompts: Nsw "Number of Ideal Switches"; Rsw "Switchr resistances"; Ts "Sample Time (s)"
  saturable_transformer : Subsystem  mask(Saturable transformer model){isat=[1,2,3,5], phisat=[1,2,3,4], fluxinit=0, Ts=50e-6}
      mask prompts: isat "Saturation current:"; phisat "Flux saturation:"; fluxinit "Initial flux:"; Ts "Sample time Ts(sec):"
      mask help:
      | Models the saturation of a three winding saturable transformer.
      |
      | The saturation characteristic should be given in increasing order starting with current-flux pair (0,0). Only positive part of the characteristic must be entered. If the initial flux parameter (phi0) is not declared, the flux will be initialized automatically according to the steady-state voltage across the magnetizing branch. Set winding no.3 parameters to zero to implement a two winding transformer.
  simplified_sync_mach : Subsystem  mask(Simplified Synchronous Machine Model){v6=4-wire Y, v1=[ 1000  120*sqrt(3/2)  60 ], v2=[ inf  0  2 ], v3=[ 1e-6  1e-6 ], v4=[ 0   0   0,0,0   0,0,0 ], v5=off, Ts=1}
      mask prompts: v6 "Connection type:"; v1 "Nom. power, L-L volt., and freq. [ Pn(VA) Vn(Vrms) fn(Hz) ]:"; v2 "Inertia, damping factor and pairs of poles[ H(s)  Kd() p() ]:"; v3 "Internal impedance [ R,X (p.u.) ]:"; v4 "Init. cond. [ dw(%)  th(deg)  ia,ib,ic(p.u.)  pha,phb,phc(deg) ]:"; v5 "I/O units (check for S.I., otherwise p.u.):"; Ts "Sample Time (s):"
      mask help:
      | Implements a 3-phase simplified synchronous machine. Machine is modelled as an internal voltage behind a R-L impedance. Stator windings are connected in wye to an internal neutral point.
      |
      | 1st input: Simulink signal:  mechanical power supplied to
      |          the machine (p.u., >0 for generator mode,
      |          <0 for motor mode)
      | 2nd input: Simulink signal: internal voltage (p.u.)
      |
      | First 3 outputs: Machine terminals = phases a, b and c
      | 4th output: Simulink measurement output = vector (12x1) containing :
      |    1-3 : Line currents flowing out of machine ia, ib, ic
      |    4-6 : Terminal voltages va, vb, vc
      |    7-9 : Internal voltages ea, eb, ec
      |    10   : Electrical angle theta
      |    11   : Rotor speed n
      |    12   : Electrical power Pe
      |
      | Units of mesurement output depend on checkbox in block's dialog box.
      mask init:
      | [Pb,Nb,Vb,Vb2,Vb3,ib,ib2,web_psb,H,Kd,p,pi23,R,L,io,dwo,tho]=powericonV2('Simplified Synchronous Machine Model',v1,v2,v3,v4,v5);
      | if v6==1,sel=1:2; else sel=1:3; end
      mask StyleString: popup(3-wire Y|4-wire Y),edit,edit,edit,edit,checkbox,edit
  surge_arrester : Subsystem  mask(Surge arrester model){uref=185e3, n=30, iref=500, param1=[.955 50], param2=[1.0 25], param3=[.9915 16.5], Ts=1}
      mask prompts: uref "Protection voltage  (V):"; n "Number of columns:"; iref "Nominal current per column  (A):"; param1 "Segment 1 characteristics: [ k1 alpha1 ]"; param2 "Segment 2 characteristics: [ k2 alpha2 ]"; param3 "Segment 3 characteristics: [ k3 alpha3 ]"; Ts "Sample Time (s)"
      mask help: The surge arrester model is a Metal oxide varistor.
      mask init: same as powerlib_modelsV2/Continuous/surge_arrester
  synchronous_machine : Subsystem  mask(Synchronous Machine Model){v1=[202000000      13800         60], v2=[0.003     0.19837     0.91763     0.21763], v3=[0.00063581     0.16537], v4=[0.0046454              0.039203              0.006843              0.014544                     0                   Inf], v5=[Inf             0            32], v6=[0  0  0  0  0  0  0  0  0], v9=off, v7=[], v10=off, Ts=1, excAxis=Field (d axis)}
      mask prompts: v1 "Nom. power, L-L volt., freq. and [field cur.] [ Pn(VA) Vn(Vrms) fn(Hz) [ifn(A)] ]:"; v2 "Stator [ Rs  Ll  Lmd  Lmq ] (pu):"; v3 "Field [ Rf  Llfd ] (pu):"; v4 "Dampers [ Rkd  Llkd  Rkq1  Llkq1  Rkq2  Llkq2 ] (pu):"; v5 "Coeff. of inertia, friction factor and pairs of poles [ H(s)  F(pu)  p() ]:"; v6 "Init. cond. [ dw(%)  th(deg)  ia,ib,ic(pu)  pha,phb,phc(deg)  Vf(pu) ]:"; v9 "Simulate saturation"; v7 "Saturation parameters [ ifd1,ifd2,... (p.u.) ; vt1,vt2,... (p.u.) ]:"; v10 "I/O units (check for S.I., otherwise p.u.):"; Ts "Sample Time (s):"; excAxis "Excitation voltage:"
      mask init:
      | if (~isempty(exist(v7)) & v9) 
      | 	sat=str2num(v7);
      | else 
      | 	sat=[]; 
      | end;
      | [Rs,Ll,Lad,Laq,Rf,Llfd,Rkd,Rkq1,Rkq2,Llkd,Llkq1,Llkq2,H,F,p,dwo,tho,phido,phikdo,phifdo,phiqo,phikq1o,phikq2o,phib,Pb,Vb,Vb2,ib,ib2,Nb,N,N2,phis,a]=powericonV2('Synchronous Machine Model',v1,v2,v3,v4,v5,v6,sat,0,v10,excAxis);
      | a5=a(1); 
      | a4=a(2); 
      | a3=a(3); 
      | a2=a(4); 
      | a1=a(5); 
      | a0=a(6); 
      | Lmd=v2(3); 
      | Lmq=v2(4);
      | web_psb=v1(3)*2*pi;
      | one_third=1/3; 
      | sqrt3=sqrt(3);
      | if v10==1
      |    Gain1 = Pb;
      | else
      |    Gain1 = 1;
      | end
      mask StyleString: edit,edit,edit,edit,edit,edit,checkbox,edit,checkbox,edit,popup(Field (d axis)|Damper 1 (q axis - used for testing only))
  thyristor (logical) : Subsystem  mask(thyristors logic model){Nsw=1, Vf=0, Rsw=1, Ts=1}
      mask prompts: Nsw "Number of thyristors"; Vf "Forward voltage Vf (V)"; Rsw "Thyristor resistances"; Ts "Sample time (s):"

== system powerlib_modelsV2/Phasors ==
  3_Phase_Prog_Source : Subsystem  mask(3-phase Programmable Source){Par_Vps_LLrms=Par_Vps, VariationEntity=None, VariationType=Step, VariationStep=VariationStep, VariationRate=VariationRate, VariationMag=VariationMag, VariationFreq=VariationFreq, Par_Timing_Variation=Par_Timing_Variation, SinglePhase=off, Yampli=Yampli, Xtime=Xtime, HarmonicGeneration=off, Par_HarmoA_pu=Par_HarmoA_pu, Par_HarmoB_pu=Par_HarmoB_pu, Par_Timing_Harmo=Par_Timing_Harmo}
      mask prompts: Par_Vps_LLrms "Positive-sequence: [ Amplitude  Phase(degrees)   Freq. (Hz) ]"; VariationEntity "Time variation of:"; VariationType "Type of variation:"; VariationStep "Step magnitude:"; VariationRate "Rate of change (value/s):"; VariationMag "Amplitude of the modulation:"; VariationFreq "Frequency of the modulation(Hz):"; Par_Timing_Variation "Variation timing (s) : [ Start   End ]"; SinglePhase "1-phase only"; Yampli "Amplitude values:"; Xtime "Time values:"; HarmonicGeneration "Harmonic generation:"; Par_HarmoA_pu "A:  [ Order(n)   Amplitude  Phase(degrees)  Seq(0, 1 or 2) ]"; Par_HarmoB_pu "B:  [ Order(n)   Amplitude  Phase(degrees)  Seq(0, 1 or 2) ]"; Par_Timing_Harmo "Harmonic timing (s) : [ Start   End ]"
      mask help: Use this block to generate a set of three-phase sinusoidal voltages or currents a, b and c. Time variation for the amplitude, phase and frequency of the fundamental can be pre-programmed. In addition, two harmonics can be surimposed on the fundamental.
      mask init:
      | % Conversion of pos. seq.amplitude from Ph-Ph rms voltage to Ph-G peak
      | Par_Vps=Par_Vps_LLrms;
      | Par_Vps(1)=Par_Vps(1)*sqrt(2/3);
      | Mag_Vps=Par_Vps(1);
      | Phase_Vps=Par_Vps(2);
      | Freq_Vps=Par_Vps(3);
      | % Conversion of harmonic amplitudes from pu to Ph-G peak volt
      | Par_HarmoA=Par_HarmoA_pu;
      | Par_HarmoB=Par_HarmoB_pu;
      | Par_HarmoA(2)=Par_HarmoA(2)*Mag_Vps;
      | Par_HarmoB(2)=Par_HarmoB(2)*Mag_Vps;
      | % Conversion of amplitude variation from pu to Ph-G peak volt
      | if VariationEntity==2
      | 	VariationStep=VariationStep*Mag_Vps;
      | 	VariationRate=VariationRate*Mag_Vps;
      | 	VariationMag=VariationMag*Mag_Vps;
      | 	Yampli=Yampli*Mag_Vps;
      | end
      | 
      | Ton_Variation=Par_Timing_Variation(1);
      | Toff_Variation=Par_Timing_Variation(2);
      | n_HarmoA=Par_HarmoA(1);
      | Mag_HarmoA=Par_HarmoA(2);
      | Phase_HarmoA=Par_HarmoA(3);
      | Seq_HarmoA=Par_HarmoA(4);
      | if n_HarmoA==0
      |     Phase_HarmoA=90;
      |     Seq_HarmoA=0;
      | end
      | n_HarmoB=Par_HarmoB(1);
      | Mag_HarmoB=Par_HarmoB(2);
      | Phase_HarmoB=Par_HarmoB(3);
      | Seq_HarmoB=Par_HarmoB(4);
      | if n_HarmoB==0
      |     Phase_HarmoB=90;
      |     Seq_HarmoB=0;
      | end
      | Ton_Harmo=Par_Timing_Harmo(1);
      | Toff_Harmo=Par_Timing_Harmo(2);
      | 
      | if Xtime(1)~=0,
      | Xtime=[0 Xtime];
      | Yampli=[0 Yampli];
      | end
      | n=length(Xtime); vec_dt= [Xtime,0] - [0,Xtime] ; vec_dt=vec_dt(2:n);
      mask StyleString: edit,popup(None|Amplitude|Phase|Frequency),popup(Step|Ramp|Modulation|Table of time-amplitude pairs),edit,edit,edit,edit,edit,checkbox,edit,edit,checkbox,edit,edit,edit
  3_phase_source : Subsystem  mask{A=1, P=0, F=60}
      mask prompts: A "Amplitude"; P "Phase (of phase A)"; F "Frequency"
  Dynamic_Load : Subsystem  mask(3-Phase Dynamic Load - Phasor Type){Vfnom=[ 500e3 60 ], PQ_0=[ 50e6 25e6], V0=[0.9844  -1.41 ], PQext=off, n=[1  1], Tpq=[0  0  0  0], Vmin=0.7, Reserved=0}
      mask prompts: Vfnom "Nominal L-L voltage and freqency  [Vn(Vrms) fn(Hz)]:"; PQ_0 "Active & reactive power at initial voltage [Po(W) Qo(var)]:"; V0 "Initial positive-sequence voltage Vo [Mag(pu) Phase (deg.)]:"; PQext "External control of PQ"; n "Parameters [ np  nq ]:"; Tpq "Time constants [Tp1 Tp2 Tq   edit     Tpq"; Vmin "Minimum voltage Vmin (pu):"
      mask help:
      | This block implements a three-phase, three-wire dynamic load whose active  power P and reactive power Q vary as function of positive-sequence voltage. Negative- and zero-sequence currents are not simulated. The three load currents are therefore balanced, even under unbalanced load voltage conditions.
      |
      |   If V>Vmin, P and Q vary as follows:
      |        P=Po*(V/Vo)^np
      |        Q=Qo*(V/Vo)^nq
      | where:
      | Po, Qo : active and reactive powers at specified voltage Vo
      |   V : positive-sequence voltage
      |   Vmin : minimum voltage below which load impedance
      |              is kept constant (np=nq=2)
      | np,nq : exponents (usually comprised between 1 and 3)
      |               controlling the nature of the load.
      | For example, specify  np=nq=1 for a constant current load; np=nq=2  for a  constant impedance load.
      |
      | Check 'External control of PQ'  to control power from a vectorized signal  [P Q] connected to input  4.
      | The m output returns a vector of 3 signals [V(pu) P(W) Q (var)].
      mask init:
      | Vnom = Vfnom(1) ; fnom=Vfnom(2);
      | P0 = PQ_0(1) ;  Q0 = PQ_0(2) ;
      | Mag_V0=V0(1); Pha_V0=V0(2);
      | V0_d=Mag_V0*cos(Pha_V0*pi/180);
      | V0_q=Mag_V0*sin(Pha_V0*pi/180);
      | np = n(1) ; nq = n(2) ;
      | Tp1=Tpq(1); Tp2=Tpq(2); Tq1=Tpq(3); Tq2=Tpq(4);
      | Vbase=Vnom/sqrt(3)*sqrt(2);
      | % initial value of positive-sequence current I1
      | a=exp(j*2*pi/3);
      | I1_init=(P0-j*Q0)/((V0_d-j*V0_q)*Vnom)/sqrt(3)*sqrt(2);
      | Mag_ia=abs(I1_init);
      | Phase_ia=angle(I1_init)*180/pi;
      mask CallbackString: |||parametres=get_param(gcb,'MaskValues');p4=parametres{4};if strcmp(p4,'on');param5='off';param6='off';param7='off';else ;param5='on';param6='on';param7='on';end;visible={'on','on','on','on',param5,param6,param7,'off'};set_param(gcb,'MaskVisibilities',visible)||||
  Impedance Measurement : Subsystem
      mask Type: Impedance Measurement model
      mask Description: Simulink model for the Impedance Measurement block. The model  injects a null current in the circuit.
  asynchronous_machine : Subsystem  mask(Asynchronous Machine Model){rotType=Squirrel-cage, ctrl=Rotor, nom=[1678500 2400 60], sta=[0.00845078125 0.0658562609861519], rot=[0.0064109375 0.0658562609861519], Lm=3.79984797902399, mec=[0.676001751311075 0 2], ini=[1 0 0 0 0 0 0 0], iounits=on}
      mask prompts: rotType "Rotor type:"; ctrl "Reference frame:"; nom "Nom. power,L-L volt. and freq. [ Pn(VA),Vn(Vrms),fn(Hz) ]:"; sta "Stator [ Rs,Lls (p.u.) ]:"; rot "Rotor [ Rr',Llr' (p.u.) ]:"; Lm "Magnetizing inductance Lm (p.u.):"; mec "Inertia constant,friction factor and pairs of poles [ H(s)  F(p.u.)  p() ]:"; ini "Initial conditions [ s()  th(deg)   isa,isb,isc(p.u.)   pha,phb,phc(deg) ]:"; iounits "I/O units (check for S.I., otherwise p.u.)"
      mask help: Implements a three-phase asynchronous machine (wound rotor or squirrel cage) modelled in the dq rotor reference frame. Stator and rotor windings are connected in wye to an internal neutral point. Press help for inputs and outputs description.
      mask init:
      | [Rs,Lls,Rr,Llr,H,F,p,Laq,Lad,web,Vb,Vb2,ib,ib2,phib2,Nb2,Tb2,phisqo,phisdo,phirqo,phirdo,wmo,tho] = powericonV2('Asynchronous Machine Model',nom, sta, rot, Lm, mec,ini,iounits);one_third=1/3; sqrt3_3=sqrt(3)/3;sqrt3=sqrt(3);
      | switch rotType
      |     case 1, selWidth=6; elements1=3:6; elements2=1:4;
      |     case 2, selWidth=4; elements1=1:4; elements2=3:4;
      | end
      mask Help: First 3 inputs: Stator terminals = phases a, b and c; 4th input: Simulink signal = Mechanical torque applied to the shaft (p.u., >0 for motor mode, <0 for generator mode); First 3 outputs: Rotor terminals = phases a, b and c; 4th output: Simulink measurement output = vector (20x1) containing the following (all currents flowing into the machine): [1-3] : Rotor line currents ira, irb and irc; [4-5] : Rotor currents iqr and idr; [6-7] : Rotor fluxes phiqr and  phidr; [8-9] : Rotor voltages vqr and vdr; [10-12] : Stator line currents isa, isb, isc; [13-14] : Stator currents iqs and ids; [15-16] : Stator fluxes phiqs and  phids; [17-18] : Stator voltages vqs and vds; [19] : Rotor speed wm; [20 ]: Electromagnetic torque Te. Units of output measurement depend on checkbox in block's dialog box.
      mask StyleString: popup(Wound|Squirrel-cage),popup(Rotor|Stationary|Synchronous),edit,edit,edit,edit,edit,edit,checkbox
  breaker : Subsystem  mask(Switch logic model){istate=0, Nsw=1, Rsw=1, Ts=0}
      mask prompts: Nsw "Number of switches"; Rsw "Breaker Resistances"
      mask help: Simulink model for the Ideal Switch block during a continuous simulation. The switching logic of the ideal switch is handled by the sfun_psbcontc.c function.
  distributed_param_line : Subsystem  mask(Distributed Parameter Line Model){nphase=3, f=60, ri=[0.01273 0.3864], li=[0.9337e-3  4.1264e-3], ci=[12.74e-9 7.751e-9], long=100, V1_init=[0 0 0 0; 0.0001244 0 0 0; 0.0002488 0 0 0; 0.0003733 0 0 0; 0.0004977 0 0 0; 0.0006221 0 0 0], V2_init=[0 0 0 0; 0.0001244 0 0 0; 0.0002488 0 0 0; 0.0003733 0 0 0; 0.0004977 0 0 0; 0.0006221 0 0 0], I1_init=[0 0 0 0; 0.0001244 0 0 0; 0.0002488 0 0 0; 0.0003733 0 0 0; 0.0004977 0 0 0; 0.0006221 0 0 0], I2_init=[0 0 0 0; 0.0001244 0 0 0; 0.0002488 0 0 0; 0.0003733 0 0 0; 0.0004977 0 0 0; 0.0006221 0 0 0], time_init=0}
      mask prompts: nphase "Number of phases"; f "Frequency used for R L C specification (Hz)"; ri "R [3*3 matrix] or [R0 R1] (ohms/km)"; li "L [3*3matrix ] or [L0 L1] (H/km)"; ci "C [3*3matrix] or [C0 C1] (F/km)"; long "Line length (km)"; time_init "time delay init"
      mask help: Simulink model for the Distributed Parameter Line block. The last five parameters are automatically calculated by SimPowerSystems at the begining of the simulation.
      mask init:
      | [Zm,R,v,Ti]=powericonV2('Distributed Parameter Line Model',nphase,f,ri,li,ci);to=long./v;Rt4=R*long/4;h=(Zm-Rt4)./(Zm+Rt4);
  ideal_switch : Subsystem  mask(Switch logic model){Nsw=1, Rsw=1, Ts=0}
      mask prompts: Nsw "Number of switches"; Rsw "Switch resistances"
      mask help: Simulink model for the Ideal Switch block during a continuous simulation. The switching logic of the ideal switch is handled by the sfun_psbcontc.c function.
  simplified_sync_mach : Subsystem  mask(Simplified Synchronous Machine Model){v6=3-wire Y, v1=[200e6 13800 60], v2=[3.6 0 2], v3=[0.02 0.2], v4=[0 18.9108 0.754635 0.754635 0.754635 16.6258 -103.374 136.626], v5=off}
      mask prompts: v6 "Connection type:"; v1 "Nom. power, L-L volt., and freq. [ Pn(VA) Vn(Vrms) fn(Hz) ]:"; v2 "Inertia, damping factor and pairs of poles[ H(s)  Kd() p() ]:"; v3 "Internal impedance [ R,X (p.u.) ]:"; v4 "Init. cond. [ dw(%)  th(deg)  ia,ib,ic(p.u.)  pha,phb,phc(deg) ]:"; v5 "I/O units (check for S.I., otherwise p.u.):"
      mask help:
      | Implements a 3-phase simplified synchronous machine. Machine is modelled as an internal voltage behind a R-L impedance. Stator windings are connected in wye to an internal neutral point.
      |
      | 1st input: Simulink signal:  mechanical power supplied to
      |          the machine (p.u., >0 for generator mode,
      |          <0 for motor mode)
      | 2nd input: Simulink signal: internal voltage (p.u.)
      |
      | First 3 outputs: Machine terminals = phases a, b and c
      | 4th output: Simulink measurement output = vector (12x1) containing :
      |    1-3 : Line currents flowing out of machine ia, ib, ic
      |    4-6 : Terminal voltages va, vb, vc
      |    7-9 : Internal voltages ea, eb, ec
      |    10   : Electrical angle theta
      |    11   : Rotor speed n
      |    12   : Electrical power Pe
      |
      | Units of mesurement output depend on checkbox in block's dialog box.
      mask init:
      | [Pb,Nb,Vb,Vb2,Vb3,ib,ib2,web,H,Kd,p,pi23,R,L,io,dwo,tho]=powericonV2('Simplified Synchronous Machine Model',v1,v2,v3,v4,v5);
      | if v6==1,sel=1:2; else sel=1:3; end
      | Id1o=v4(3)*cos(v4(6)*pi/180);
      | Iq1o=v4(3)*sin(v4(6)*pi/180);
      mask StyleString: popup(3-wire Y|4-wire Y),edit,edit,edit,edit,checkbox
  synchronous_machine : Subsystem  mask(Synchronous Machine Model){v1=[3125000 2400 60], v2=[0.0036 0.0311592623858907 1.52884073761411 1.02884073761411], v3=[0.000252115160438864 0.321093931414665], v4=[0.0186554012805331 0.323797404426229 0.0635966848600831 0.169928530080505 0 Inf], v5=[1.07 0 2], v6=[0 -114.435 0.362123 0.362123 0.362123 -95.3524 144.648 24.6476 1.52654], v9=off, v7=0, v10=off, excAxis=Field (d axis)}
      mask prompts: v1 "Nom. power, L-L volt., freq. and [field cur.] [ Pn(VA) Vn(Vrms) fn(Hz) [ifn(A)] ]:"; v2 "Stator [ Rs  Ll  Lmd  Lmq ] (pu):"; v3 "Field [ Rf  Llfd ] (pu):"; v4 "Dampers [ Rkd  Llkd  Rkq1  Llkq1  Rkq2  Llkq2 ] (pu):"; v5 "Coeff. of inertia, friction factor and pairs of poles [ H(s)  F(pu)  p() ]:"; v6 "Init. cond. [ dw(%)  th(deg)  ia,ib,ic(pu)  pha,phb,phc(deg)  Vf(pu) ]:"; v9 "Simulate saturation"; v7 "Saturation parameters [ ifd1,ifd2,... (p.u.) ; vt1,vt2,... (p.u.) ]:"; v10 "I/O units (check for S.I., otherwise p.u.):"; excAxis "Excitation voltage:"
      mask init:
      | if (~isempty(exist(v7)) & v9) sat=str2num(v7);else sat=[]; end;
      | [Rs,Ll,Lad,Laq,Rf,Llfd,Rkd,Rkq1,Rkq2,Llkd,Llkq1,Llkq2,H,F,p,dwo,tho,phido,phikdo,phifdo,phiqo,phikq1o,phikq2o,phib,Pb,Vb,Vb2,ib,ib2,Nb,N,N2,phis,a]=powericonV2('Synchronous Machine Model',v1,v2,v3,v4,v5,v6,sat,0,v10,excAxis);
      | a5=a(1); a4=a(2); a3=a(3); a2=a(4); a1=a(5); a0=a(6); Lmd=v2(3); Lmq=v2(4);
      | web=v1(3)*2*pi; one_third=1/3; sqrt3=sqrt(3);
      | 
      | % Computation of negative sequence impedance
      | %  L"d= Ll +1/(1/Lmd +1/Llfd + 1/Llkd)
      |  Lsecd=v2(2)+1/(1/v2(3)+1/v3(2)+1/v4(2));
      | %  L"q= Ll +1/(1/Lmq +1/Llkq1 + 1/Llkq2)
      | Lsecq=v2(2)+1/(1/v2(4)+1/v4(4)+1/v4(6));
      | %L2=2(L"d*L"q/(L"d+L"q) (Kundur p881)
      | L2_pu=2*(Lsecd*Lsecq/(Lsecd+Lsecq));
      | 
      | % initial values of Id Iq:  Idqo= mag(Ia) <( phi(Ia-)-thetao))
      | Idqo=v6(3)*exp(j*(v6(6)-v6(2))*pi/180);
      | Ido=real(Idqo); Iqo=imag(Idqo);
      | 
      | if strcmp('on',v10)
      |    Gain1 = 3/2;
      | else
      |    Gain1 = 1;
      | end
      mask StyleString: edit,edit,edit,edit,edit,edit,checkbox,edit,checkbox,popup(Field (d axis)|Damper 1 (q axis - used for testing only))
